simulink model "Semi_Active_Road_Profile_2"  (R2017b)
settings: Solver=VariableStepAuto  StartTime=0.0  StopTime=40  RelTol=1e-3
undefined symbols (not defined in the file): sigbuilder_block
settings Model: SimulationMode=accelerator  Creator=LENOVO  LastModifiedBy=LENOVO
settings DebuggingCC: MaxConsecutiveZCsMsg=none

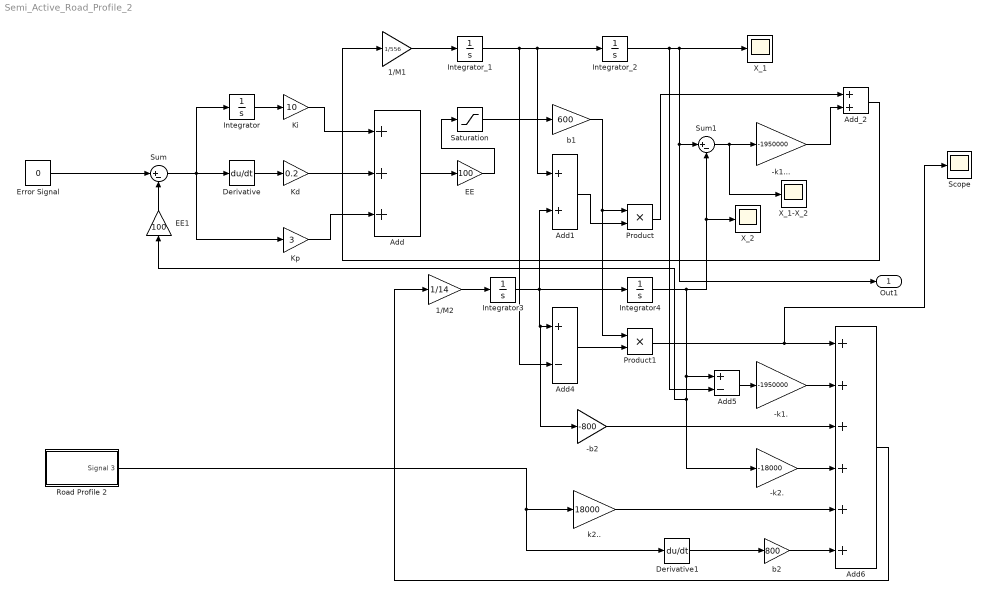
== system Semi_Active_Road_Profile_2 ==
  -b2 : Gain  Gain=-800
  -k1. : Gain  Gain=-1950000
  -k1... : Gain  Gain=-1950000
  -k2. : Gain  Gain=-18000
  1/M1 : Gain  Gain=1/556
  1/M2 : Gain  Gain=1/14
  "Add " : Sum  Inputs=+++
  "Add1 " : Sum
  "Add4 " : Sum  Inputs=+-
  Add5 : Sum  Inputs=+-
  Add6 : Sum  Inputs=++++++
  Add_2 : Sum
  "Derivative " : Derivative
  Derivative1 : Derivative
  EE : Gain  Gain=100
  EE1 : Gain  Gain=100
  Error Signal : Constant  Value=0
  "Integrator " : Integrator
  Integrator3 : Integrator
  Integrator4 : Integrator
  "Integrator_1 " : Integrator
  "Integrator_2 " : Integrator
  Kd : Gain  Gain=0.2
  Ki : Gain  Gain=10
  Kp : Gain  Gain=3
  "Product " : Product
  Product1 : Product
  Road Profile 2 : Subsystem  Tag=STV Subsys  LoadFcn=sigbuilder_block('load');  StartFcn=sigbuilder_block('start');  StopFcn=sigbuilder_block('stop');  ClipboardFcn=sigbuilder_block('clipboard');  mask(Sigbuilder block){tuvar=[0:10]}
      mask help: Simulink:masks:SigbuilderBlock_MD
      mask init:
      | if ~strcmp(get_param(bdroot(gcbh),'SimulationStatus'),'stopped') tuvar = sigbuilder_block('maskInit'); end
      settings: CopyFcn=sigbuilder_block('copy');  DeleteFcn=sigbuilder_block('delete');  ModelCloseFcn=sigbuilder_block('modelClose');  PreSaveFcn=sigbuilder_block('preSave');  PauseFcn=sigbuilder_block('pause');  ContinueFcn=sigbuilder_block('continue');  NameChangeFcn=sigbuilder_block('namechange');  OpenFcn=sigbuilder_block('open',[141 130.5 550.5 359.25 ]);  CloseFcn=sigbuilder_block('close');
      mask Display: plot(0, 0, 100, 100,[2, 2, 32, 32, 2], [68, 8, 8, 68, 68],[32, 2], [38, 38], [32, 19, 2],[53, 60, 44], [32, 17, 17, 2],[16, 16, 31, 31]);txt = getActiveGroup(gcbh);text(2, 100, txt,'verticalAlignment', 'top');
  Saturation : Saturate  UpperLimit=1  LowerLimit=-1
  Scope : Scope
  Sum : Sum  Inputs=|+-
  Sum1 : Sum  Inputs=|+-
  X_1 : Scope
  X_1-X_2 : Scope
  X_2 : Scope
  b1 : Gain  Gain=600
  b2 : Gain  Gain=800
  k2.. : Gain  Gain=18000
  Out1 : Outport
  wires:
  "Integrator "/1 -> Ki/1
  "Derivative "/1 -> Kd/1
  Kp/1 -> "Add "/3
  Kd/1 -> "Add "/2
  Ki/1 -> "Add "/1
  Sum/1 -> Kp/1, "Integrator "/1, "Derivative "/1
  "Add "/1 -> EE/1
  EE/1 -> Saturation/1
  Saturation/1 -> b1/1
  1/M1/1 -> "Integrator_1 "/1
  "Integrator_1 "/1 -> "Add4 "/2, "Add1 "/1, "Integrator_2 "/1
  "Integrator_2 "/1 -> Add5/2, X_1/1, Sum1/1, Out1/1
  -k1.../1 -> Add_2/2
  Sum1/1 -> -k1.../1, X_1-X_2/1
  1/M2/1 -> Integrator3/1
  Integrator4/1 -> X_2/1, Sum1/2, Add5/1, EE1/1, -k2./1
  Integrator3/1 -> "Add1 "/2, Integrator4/1, -b2/1, "Add4 "/1
  "Add4 "/1 -> Product1/2
  b1/1 -> "Product "/1, Product1/1
  Add_2/1 -> 1/M1/1
  Product1/1 -> Scope/1, Add6/1
  -k1./1 -> Add6/2
  Add5/1 -> -k1./1
  -k2./1 -> Add6/4
  -b2/1 -> Add6/3
  "Add1 "/1 -> "Product "/2
  Derivative1/1 -> b2/1
  b2/1 -> Add6/6
  k2../1 -> Add6/5
  Road Profile 2/1(Signal 3) -> k2../1, Derivative1/1
  "Product "/1 -> Add_2/1
  Add6/1 -> 1/M2/1
  Error Signal/1 -> Sum/1
  EE1/1 -> Sum/2

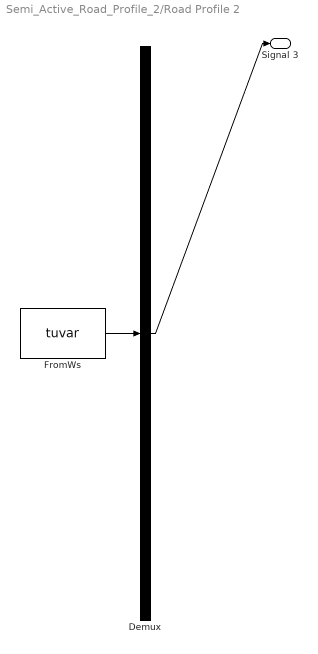
== system Semi_Active_Road_Profile_2/Road Profile 2 ==
  Demux : Demux  Tag=STV Demux  Outputs=1
  FromWs : FromWorkspace  Tag=STV FromWs  VariableName=tuvar  SampleTime=0
      SigBuilderData=|
      | common.afterFinalStr = 'Extrapolate'
      | common.sampleTime = 0
      | dataSet.timeRange = [0 40]
      | dataSet.name = 'Group 1'
      | sbobj.Groups.Name = 'Group 1'
      | sbobj.Groups.Signals.Name = 'Signal 3'
      | sbobj.Groups.Signals.XData = [0 5 5 40]
      | sbobj.Groups.Signals.YData = [0 0 0.1 0.1]
      | sbobj.Groups.TimeRange = [0 40]
  Signal 3 : Outport  Tag=STV Outport
  wires:
  FromWs/1 -> Demux/1
  Demux/1 -> Signal 3/1
